simulink model "Cascaded_Filter"  (R2020a)
settings: Solver=VariableStepAuto  StartTime=0.0  StopTime=10.0  RelTol=1e-3
settings Model: Creator=kasutav  LastModifiedBy=kasutav
settings DataIOCC: SaveOutput=off  SaveTime=off

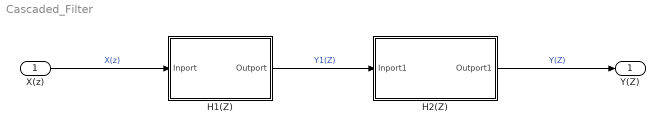
== system Cascaded_Filter ==
  X(z) : Inport  OutDataTypeStr=double  PortDimensions=1  SampleTime=[0,1]
  H1(Z) : Subsystem
  H2(Z) : Subsystem
  Y(Z) : Outport  OutDataTypeStr=double  PortDimensions=1  SampleTime=[0,1]
  wires:
  H2(Z)/1(Outport1) -> Y(Z)/1  "Y(Z)"
  X(z)/1 -> H1(Z)/1(Inport)  "X(z)"
  H1(Z)/1(Outport) -> H2(Z)/1(Inport1)  "Y1(Z)"

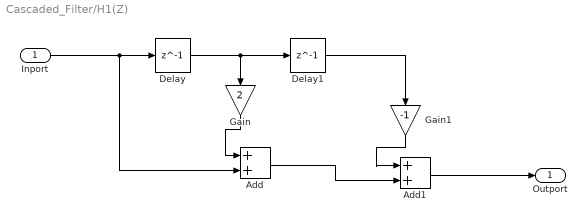
== system Cascaded_Filter/H1(Z) ==
  Inport : Inport
  Add : Sum
  Add1 : Sum
  Delay : Delay  DelayLength=1
  Delay1 : Delay  DelayLength=1
  Gain : Gain  Gain=2
  Gain1 : Gain  Gain=-1
  Outport : Outport
  wires:
  Delay/1 -> Delay1/1, Gain/1
  Add/1 -> Add1/2
  Inport/1 -> Delay/1, Add/2
  Delay1/1 -> Gain1/1
  Gain1/1 -> Add1/1
  Add1/1 -> Outport/1
  Gain/1 -> Add/1

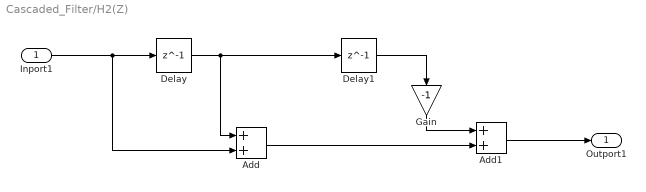
== system Cascaded_Filter/H2(Z) ==
  Inport1 : Inport
  Add : Sum
  Add1 : Sum
  Delay : Delay  DelayLength=1
  Delay1 : Delay  DelayLength=1
  Gain : Gain  Gain=-1
  Outport1 : Outport
  wires:
  Delay1/1 -> Gain/1
  Delay/1 -> Delay1/1, Add/1
  Inport1/1 -> Delay/1, Add/2
  Gain/1 -> Add1/1
  Add1/1 -> Outport1/1
  Add/1 -> Add1/2
